simulink model "PVHome"  (R2022b)
settings: Solver=FixedStepDiscrete  StartTime=0.0  StopTime=2  FixedStep=5e-6  RelTol=1e-3
undefined symbols (not defined in the file): Ion, Lithium
libraries: spsSeriesRLCBranchLib x175, spsBreakerLib x103, spsPWMGeneratorDCDCLib x94, spsThyristorLib x78, slpidlib x72, spsIGBTDiodeLib x62, spsThreePhaseVIMeasurementLib x59, spsThreePhaseBreakerLib x45, spsVoltageMeasurementLib x45, spsDiodeLib x39, spsThreePhaseParallelRLCBranchLib x38, spsMosfetLib x32
(part 15 of 16)

== matlab function PVHome/Subsystem6/Centralized System ==
  data: H1_Pv_Breaker output; P_Pv input; Bi_B_Charge_Breaker_Buck output; Bi_B_Charge_Breaker_Boost output; H1_Grid_Breaker output; H1_Grid_Circuit_Breaker output; P_load input; Bi_B_Breaker_Discharge_Boost output; Bi_B_Breaker_Discharge_Buck output; H1_B_Ground_Discharge output; SOCbH1 input; Grid_Energy_Trading_Breaker output; Wind_Breaker_Boost output; P_Wind input; P_Real_Grid input; Wind_Breaker_Buck output; V_PV_1 input; V_Wind input; Wind_Power_Battery_Breaker_Boost output; Wind_Power_Battery_Breaker_Buck output; Battery_Passing_Voltage input; P1_C1 output
function [H1_Pv_Breaker, Bi_B_Charge_Breaker_Buck,Bi_B_Charge_Breaker_Boost, H1_Grid_Breaker, H1_Grid_Circuit_Breaker,Bi_B_Breaker_Discharge_Boost, Bi_B_Breaker_Discharge_Buck, H1_B_Ground_Discharge, Grid_Energy_Trading_Breaker, Wind_Breaker_Boost, Wind_Breaker_Buck, Wind_Power_Battery_Breaker_Boost, Wind_Power_Battery_Breaker_Buck, P1_C1] = control_logic(P_Pv, P_load, SOCbH1, P_Wind, P_Real_Grid, V_PV_1, V_Wind, Battery_Passing_Voltage)

% Make positive
P_Pv   = abs(P_Pv);
P_load = abs(P_load);
SOCbH1 = abs(SOCbH1);
P_Wind = abs(P_Wind);
V_PV_1 = abs(V_PV_1);
V_Wind = abs(V_Wind);
Battery_Passing_Voltage = abs(Battery_Passing_Voltage);

eps = 1;

%% DEFAULT STATES

% DC Ideal Switches (1 = ON)
H1_Pv_Breaker = 0;
Bi_B_Charge_Breaker_Buck  = 0;
Bi_B_Charge_Breaker_Boost=0;
Bi_B_Breaker_Discharge_Boost=0;
Bi_B_Breaker_Discharge_Buck=0;
H1_B_Ground_Discharge=0;
Wind_Breaker_Boost=0;
Wind_Breaker_Buck=0;
Wind_Power_Battery_Breaker_Boost=0;
Wind_Power_Battery_Breaker_Buck=0;
P1_C1=0;

% AC Breakers (0 = CLOSED)
H1_Grid_Breaker = 1;  % default OPEN
H1_Grid_Circuit_Breaker = 1;  % default OPEN
Grid_Energy_Trading_Breaker=1; % default open



%% CASE 1: No PV and no Wind
if (P_Pv+ P_Wind) <= eps %eps=0.01 (almost 0)

    % DC OFF
    H1_Pv_Breaker = 0;
    Bi_B_Charge_Breaker_Buck  = 0;
    Bi_B_Breaker_Discharge_Boost=0;
    H1_B_Ground_Discharge=0;
    Bi_B_Breaker_Discharge_Buck=0;
    Wind_Breaker_Boost=0;
    Wind_Breaker_Buck=0;
    Wind_Power_Battery_Breaker_Boost=0;
    Wind_Power_Battery_Breaker_Buck=0;
    P1_C1=0;


    % AC CLOSED (use grid)
    H1_Grid_Breaker         = 0;
    H1_Grid_Circuit_Breaker = 1;
    Grid_Energy_Trading_Breaker=1; %energy trading window open


%% CASE 2: PV and wind > Load
elseif (P_Pv + P_Wind) > P_load

    % Use PV
    H1_Pv_Breaker = 1;
    H1_Grid_Breaker = 1;
    H1_Grid_Circuit_Breaker = 1;

    if (SOCbH1) < 90 % if the value of soc is between is less than 90%, the battery can charge
        
        Bi_B_Breaker_Discharge_Boost=0;
        Bi_B_Breaker_Discharge_Buck=0;
        H1_B_Ground_Discharge=0;
        Grid_Energy_Trading_Breaker=1;
        P1_C1=0;        

        if (V_PV_1 > V_Wind) %boosts up
            Wind_Power_Battery_Breaker_Boost=1;
            Wind_Power_Battery_Breaker_Buck=0;
            Wind_Breaker_Boost=1;
            Wind_Breaker_Buck=0;
            if (Battery_Passing_Voltage)>60
                Bi_B_Charge_Breaker_Buck=1;
                Bi_B_Charge_Breaker_Boost=0;
            elseif (Battery_Passing_Voltage<60)
                Bi_B_Charge_Breaker_Buck=0;
                Bi_B_Charge_Breaker_Boost=1;
            end

        elseif (V_PV_1 < V_Wind)
            Wind_Power_Battery_Breaker_Boost=0;
            Wind_Power_Battery_Breaker_Buck=1;
            Wind_Breaker_Boost=0;
            Wind_Breaker_Buck=1;
        
            if (Battery_Passing_Voltage)>60
                Bi_B_Charge_Breaker_Buck=1;
                Bi_B_Charge_Breaker_Boost=0;
            elseif (Battery_Passing_Voltage)<60
                Bi_B_Charge_Breaker_Buck=0;
                Bi_B_Charge_Breaker_Boost=1;
            end
        
        end

    elseif SOCbH1==90
        Bi_B_Charge_Breaker_Boost=0;
        Bi_B_Charge_Breaker_Buck = 0;
        Bi_B_Breaker_Discharge_Boost=0;
        Bi_B_Breaker_Discharge_Buck=0;
        H1_B_Ground_Discharge=0;
        Grid_Energy_Trading_Breaker=0; %the power is sold to grid
        P1_C1=1; %the power is sold to C1

        if (V_PV_1 > V_Wind) %boosts up
        Wind_Power_Battery_Breaker_Boost=1;
        Wind_Power_Battery_Breaker_Buck=0;
        Wind_Breaker_Boost=1;
        Wind_Breaker_Buck=0;
        if (Battery_Passing_Voltage)>60
            Bi_B_Charge_Breaker_Buck=1;
            Bi_B_Charge_Breaker_Boost=0;
        elseif (Battery_Passing_Voltage<60)
            Bi_B_Charge_Breaker_Buck=0;
            Bi_B_Charge_Breaker_Boost=1;
        end

    elseif (V_PV_1 < V_Wind)
        Wind_Power_Battery_Breaker_Boost=0;
        Wind_Power_Battery_Breaker_Buck=1;
        Wind_Breaker_Boost=0;
        Wind_Breaker_Buck=1;
        
        if (Battery_Passing_Voltage)>60
            Bi_B_Charge_Breaker_Buck=1;
            Bi_B_Charge_Breaker_Boost=0;
        elseif (Battery_Passing_Voltage)<60
            Bi_B_Charge_Breaker_Buck=0;
            Bi_B_Charge_Breaker_Boost=1;
        end
        end
    end



%% CASE 3: PV and wind < Load
elseif (P_Pv + P_Wind) < (P_load) && (H1_Grid_Breaker~=0) %open (1 means open)

    % Use PV
    H1_Pv_Breaker = 1;
    H1_Grid_Circuit_Breaker = 0;
    Grid_Energy_Trading_Breaker=1;      
    Bi_B_Charge_Breaker_Buck=0; %no charging
    Bi_B_Charge_Breaker_Boost=0; %no charging
    P1_C1=0;


    if (V_PV_1)>60
        Bi_B_Breaker_Discharge_Boost=1;
        Bi_B_Breaker_Discharge_Buck=0;
        H1_B_Ground_Discharge=1;
    elseif(V_PV_1)<60
        Bi_B_Breaker_Discharge_Boost=0;
        Bi_B_Breaker_Discharge_Buck=1;
        H1_B_Ground_Discharge=1;
    end

    if (V_PV_1 > V_Wind) %boosts up
        Wind_Power_Battery_Breaker_Boost=1;
        Wind_Power_Battery_Breaker_Buck=0;
        Wind_Breaker_Boost=1;
        Wind_Breaker_Buck=0;
        
    elseif (V_PV_1 < V_Wind)
        Wind_Power_Battery_Breaker_Boost=0;
        Wind_Power_Battery_Breaker_Buck=1;
        Wind_Breaker_Boost=0;
        Wind_Breaker_Buck=1;
    end 

    
   

           
%% CASE 4:
elseif (P_Pv + P_Wind) < (P_load) && (H1_Grid_Breaker~=1) %closed (0) (no charging)

        % Use PV
    H1_Pv_Breaker = 1;
    H1_Grid_Circuit_Breaker = 0;
    Grid_Energy_Trading_Breaker=1;      
    Bi_B_Charge_Breaker_Buck=0; %(no charging)
    Bi_B_Charge_Breaker_Boost=0; %(no charging)
    Bi_B_Breaker_Discharge_Boost=0;
    Bi_B_Breaker_Discharge_Buck=0;
    H1_B_Ground_Discharge=0;
    P1_C1=0;


    if (V_PV_1 > V_Wind) %boosts up
        Wind_Power_Battery_Breaker_Boost=1;
        Wind_Power_Battery_Breaker_Buck=0;
        Wind_Breaker_Boost=1;
        Wind_Breaker_Buck=0;
        
    elseif (V_PV_1 < V_Wind)
        Wind_Power_Battery_Breaker_Boost=0;
        Wind_Power_Battery_Breaker_Buck=1;
        Wind_Breaker_Boost=0;
        Wind_Breaker_Buck=1;
    end 


%% CASE 5:
elseif (P_Pv + P_Wind+ P_Real_Grid) < P_Load 
    % Use PV
    H1_Grid_Breaker=0;
    H1_Pv_Breaker = 1;
    H1_Grid_Circuit_Breaker = 0;
    Grid_Energy_Trading_Breaker=1;      
    Bi_B_Charge_Breaker_Buck=0; %(no charging)
    Bi_B_Charge_Breaker_Boost=0; %(no charging)
    P1_C1=0;

    %discharging
    if (V_PV_1)>60
        Bi_B_Breaker_Discharge_Boost=1;
        Bi_B_Breaker_Discharge_Buck=0;
        H1_B_Ground_Discharge=1;
    elseif(V_PV_1)<60
        Bi_B_Breaker_Discharge_Boost=0;
        Bi_B_Breaker_Discharge_Buck=1;
        H1_B_Ground_Discharge=1;
    end

    if (V_PV_1 > V_Wind) %boosts up
        Wind_Power_Battery_Breaker_Boost=1;
        Wind_Power_Battery_Breaker_Buck=0;
        Wind_Breaker_Boost=1;
        Wind_Breaker_Buck=0;
        
    elseif (V_PV_1 < V_Wind) %bucks down
        Wind_Power_Battery_Breaker_Boost=0;
        Wind_Power_Battery_Breaker_Buck=1;
        Wind_Breaker_Boost=0;
        Wind_Breaker_Buck=1;
    end 

end


end

== matlab function PVHome/Subsystem5/MATLAB Function9 ==
  data: V_PV_1 input; Wind_Breaker_Boost_Signal_Out output; Sixty input
function Wind_Breaker_Boost_Signal_Out = fcn(V_PV_1, Sixty)
V_PV_1 = abs(V_PV_1);
Sixty = abs(Sixty);

D=1-(V_PV_1/Sixty);
Wind_Breaker_Boost_Signal_Out = D; %Vout

== matlab function PVHome/Subsystem4/MATLAB Function2 ==
  data: x input; a output; ma input; shift_k input; b output; c output
function [a,b,c]=ref_generation(x,ma,shift_k)
a=(ma*(sin((x)+shift_k)));
b=(ma*(sin((x)+shift_k-(2*pi/3))));
c=(ma*(sin((x)+shift_k+(2*pi/3))));

%ma is modulation index
%x is wt rad/s
%shift_k is phase angle

== matlab function PVHome/Subsystem4/MATLAB Function3 ==
  data: u input; y output
function y = fcn(u)
% This will output 1 - u
y = 1 - u;

== matlab function PVHome/Subsystem4/MATLAB Function4 ==
  data: u input; y output
function y = fcn(u)
% This will output 1 - u
y = 1 - u;

== matlab function PVHome/Subsystem4/MATLAB Function6 ==
  data: u input; y output
function y = fcn(u)
% This will output 1 - u
y = 1 - u;

== matlab function PVHome/Subsystem4/MATLAB Function7 ==
  data: V_PV_1 input; Wind_Breaker_Boost_Signal_Out output; V_Wind input
function Wind_Breaker_Boost_Signal_Out = fcn(V_PV_1, V_Wind)
V_PV_1 = abs(V_PV_1);
V_Wind = abs(V_Wind);

D=1-(V_PV_1/V_Wind);
Wind_Breaker_Boost_Signal_Out = D; %Vout

== matlab function PVHome/Subsystem4/MATLAB Function8 ==
  data: Sixty input; Wind_Breaker_Boost_Signal_Out output; V_PV_1 input
function Wind_Breaker_Boost_Signal_Out = fcn(Sixty, V_PV_1)
Sixty = abs(Sixty);
V_PV_1 = abs(V_PV_1);

D=1-(Sixty/V_PV_1);
Wind_Breaker_Boost_Signal_Out = D; %Vout

== matlab function PVHome/Subsystem4/MATLAB Function9 ==
  data: V_PV_1 input; Wind_Breaker_Boost_Signal_Out output; Sixty input
function Wind_Breaker_Boost_Signal_Out = fcn(V_PV_1, Sixty)
V_PV_1 = abs(V_PV_1);
Sixty = abs(Sixty);

D=1-(V_PV_1/Sixty);
Wind_Breaker_Boost_Signal_Out = D; %Vout

== matlab function PVHome/Subsystem6/MATLAB Function2 ==
  data: x input; a output; ma input; shift_k input; b output; c output
function [a,b,c]=ref_generation(x,ma,shift_k)
a=(ma*(sin((x)+shift_k)));
b=(ma*(sin((x)+shift_k-(2*pi/3))));
c=(ma*(sin((x)+shift_k+(2*pi/3))));

%ma is modulation index
%x is wt rad/s
%shift_k is phase angle

== matlab function PVHome/Subsystem6/MATLAB Function3 ==
  data: u input; y output
function y = fcn(u)
% This will output 1 - u
y = 1 - u;

== matlab function PVHome/Subsystem6/MATLAB Function4 ==
  data: u input; y output
function y = fcn(u)
% This will output 1 - u
y = 1 - u;

== matlab function PVHome/Subsystem6/MATLAB Function6 ==
  data: u input; y output
function y = fcn(u)
% This will output 1 - u
y = 1 - u;

== matlab function PVHome/Subsystem6/MATLAB Function7 ==
  data: V_PV_1 input; Wind_Breaker_Boost_Signal_Out output; V_Wind input
function Wind_Breaker_Boost_Signal_Out = fcn(V_PV_1, V_Wind)
V_PV_1 = abs(V_PV_1);
V_Wind = abs(V_Wind);

D=1-(V_PV_1/V_Wind);
Wind_Breaker_Boost_Signal_Out = D; %Vout

== matlab function PVHome/Subsystem6/MATLAB Function8 ==
  data: Sixty input; Wind_Breaker_Boost_Signal_Out output; V_PV_1 input
function Wind_Breaker_Boost_Signal_Out = fcn(Sixty, V_PV_1)
Sixty = abs(Sixty);
V_PV_1 = abs(V_PV_1);

D=1-(Sixty/V_PV_1);
Wind_Breaker_Boost_Signal_Out = D; %Vout

== matlab function PVHome/Subsystem6/MATLAB Function9 ==
  data: V_PV_1 input; Wind_Breaker_Boost_Signal_Out output; Sixty input
function Wind_Breaker_Boost_Signal_Out = fcn(V_PV_1, Sixty)
V_PV_1 = abs(V_PV_1);
Sixty = abs(Sixty);

D=1-(V_PV_1/Sixty);
Wind_Breaker_Boost_Signal_Out = D; %Vout

== matlab function PVHome/Subsystem3/MATLAB Function2 ==
  data: x input; a output; ma input; shift_k input; b output; c output
function [a,b,c]=ref_generation(x,ma,shift_k)
a=(ma*(sin((x)+shift_k)));
b=(ma*(sin((x)+shift_k-(2*pi/3))));
c=(ma*(sin((x)+shift_k+(2*pi/3))));

%ma is modulation index
%x is wt rad/s
%shift_k is phase angle

== matlab function PVHome/Subsystem3/MATLAB Function3 ==
  data: u input; y output
function y = fcn(u)
% This will output 1 - u
y = 1 - u;

== matlab function PVHome/Subsystem3/MATLAB Function4 ==
  data: u input; y output
function y = fcn(u)
% This will output 1 - u
y = 1 - u;

== matlab function PVHome/Subsystem3/MATLAB Function6 ==
  data: u input; y output
function y = fcn(u)
% This will output 1 - u
y = 1 - u;

== matlab function PVHome/Subsystem3/MATLAB Function7 ==
  data: V_PV_1 input; Wind_Breaker_Boost_Signal_Out output; V_Wind input
function Wind_Breaker_Boost_Signal_Out = fcn(V_PV_1, V_Wind)
V_PV_1 = abs(V_PV_1);
V_Wind = abs(V_Wind);

D=1-(V_PV_1/V_Wind);
Wind_Breaker_Boost_Signal_Out = D; %Vout

== matlab function PVHome/Subsystem3/MATLAB Function8 ==
  data: Sixty input; Wind_Breaker_Boost_Signal_Out output; V_PV_1 input
function Wind_Breaker_Boost_Signal_Out = fcn(Sixty, V_PV_1)
Sixty = abs(Sixty);
V_PV_1 = abs(V_PV_1);

D=1-(Sixty/V_PV_1);
Wind_Breaker_Boost_Signal_Out = D; %Vout

== matlab function PVHome/Subsystem3/MATLAB Function9 ==
  data: V_PV_1 input; Wind_Breaker_Boost_Signal_Out output; Sixty input
function Wind_Breaker_Boost_Signal_Out = fcn(V_PV_1, Sixty)
V_PV_1 = abs(V_PV_1);
Sixty = abs(Sixty);

D=1-(V_PV_1/Sixty);
Wind_Breaker_Boost_Signal_Out = D; %Vout

== matlab function PVHome/Subsystem1/MATLAB Function2 ==
  data: x input; a output; ma input; shift_k input; b output; c output
function [a,b,c]=ref_generation(x,ma,shift_k)
a=(ma*(sin((x)+shift_k)));
b=(ma*(sin((x)+shift_k-(2*pi/3))));
c=(ma*(sin((x)+shift_k+(2*pi/3))));

%ma is modulation index
%x is wt rad/s
%shift_k is phase angle

== matlab function PVHome/Subsystem1/MATLAB Function3 ==
  data: u input; y output
function y = fcn(u)
% This will output 1 - u
y = 1 - u;

== matlab function PVHome/Subsystem1/MATLAB Function4 ==
  data: u input; y output
function y = fcn(u)
% This will output 1 - u
y = 1 - u;

== matlab function PVHome/Subsystem1/MATLAB Function6 ==
  data: u input; y output
function y = fcn(u)
% This will output 1 - u
y = 1 - u;

== matlab function PVHome/Subsystem1/MATLAB Function7 ==
  data: V_PV_1 input; Wind_Breaker_Boost_Signal_Out output; V_Wind input
function Wind_Breaker_Boost_Signal_Out = fcn(V_PV_1, V_Wind)
V_PV_1 = abs(V_PV_1);
V_Wind = abs(V_Wind);

D=1-(V_PV_1/V_Wind);
Wind_Breaker_Boost_Signal_Out = D; %Vout

== matlab function PVHome/Subsystem1/MATLAB Function8 ==
  data: Sixty input; Wind_Breaker_Boost_Signal_Out output; V_PV_1 input
function Wind_Breaker_Boost_Signal_Out = fcn(Sixty, V_PV_1)
Sixty = abs(Sixty);
V_PV_1 = abs(V_PV_1);

D=1-(Sixty/V_PV_1);
Wind_Breaker_Boost_Signal_Out = D; %Vout

== matlab function PVHome/Subsystem1/MATLAB Function9 ==
  data: V_PV_1 input; Wind_Breaker_Boost_Signal_Out output; Sixty input
function Wind_Breaker_Boost_Signal_Out = fcn(V_PV_1, Sixty)
V_PV_1 = abs(V_PV_1);
Sixty = abs(Sixty);

D=1-(V_PV_1/Sixty);
Wind_Breaker_Boost_Signal_Out = D; %Vout

== matlab function PVHome/Subsystem2/MATLAB Function4 ==
  data: u input; y output
function y = fcn(u)
% This will output 1 - u
y = 1 - u;

== matlab function PVHome/Subsystem2/MATLAB Function6 ==
  data: u input; y output
function y = fcn(u)
% This will output 1 - u
y = 1 - u;

== matlab function PVHome/Subsystem2/MATLAB Function7 ==
  data: V_PV_1 input; Wind_Breaker_Boost_Signal_Out output; V_Wind input
function Wind_Breaker_Boost_Signal_Out = fcn(V_PV_1, V_Wind)
V_PV_1 = abs(V_PV_1);
V_Wind = abs(V_Wind);

D=1-(V_PV_1/V_Wind);
Wind_Breaker_Boost_Signal_Out = D; %Vout

== matlab function PVHome/Subsystem2/MATLAB Function8 ==
  data: Sixty input; Wind_Breaker_Boost_Signal_Out output; V_PV_1 input
function Wind_Breaker_Boost_Signal_Out = fcn(Sixty, V_PV_1)
Sixty = abs(Sixty);
V_PV_1 = abs(V_PV_1);

D=1-(Sixty/V_PV_1);
Wind_Breaker_Boost_Signal_Out = D; %Vout

== matlab function PVHome/Subsystem2/MATLAB Function9 ==
  data: V_PV_1 input; Wind_Breaker_Boost_Signal_Out output; Sixty input
function Wind_Breaker_Boost_Signal_Out = fcn(V_PV_1, Sixty)
V_PV_1 = abs(V_PV_1);
Sixty = abs(Sixty);

D=1-(V_PV_1/Sixty);
Wind_Breaker_Boost_Signal_Out = D; %Vout

== matlab function PVHome/Subsystem6/MATLAB Function ==
  data: V_PV input; duty output; I_PV input; deltaD input
function duty = mppt_pno(V_PV, I_PV, deltaD)

persistent prevP prevDuty

if isempty(prevP)
    prevP = 0;
    prevDuty = 0.5;   % Start at 50%
end

% Current PV power
P = V_PV * I_PV;

% Basic P&O
if P > prevP
    prevDuty = prevDuty + deltaD;
else
    prevDuty = prevDuty - deltaD;
end

% Safe duty limits for boost converter
if prevDuty > 0.75
    prevDuty = 0.75;
elseif prevDuty < 0.10
    prevDuty = 0.10;
end

% Update previous power
prevP = P;

% Output duty
duty = prevDuty;

end

== matlab function PVHome/Subsystem2/MATLAB Local MPPT 2 ==
  data: V_PV_2 input; duty output; I_PV_2 input; deltaD_2 input
function duty = mppt_pno(V_PV_2, I_PV_2, deltaD_2)

persistent prevP prevDuty

if isempty(prevP)
    prevP = 0;
    prevDuty = 0.5;   % Start at 50%
end

% Current PV power
P = V_PV_2 * I_PV_2;

% Basic P&O
if P > prevP
    prevDuty = prevDuty + deltaD_2;
else
    prevDuty = prevDuty - deltaD_2;
end

% Safe duty limits for boost converter
if prevDuty > 0.75
    prevDuty = 0.75;
elseif prevDuty < 0.10
    prevDuty = 0.10;
end

% Update previous power
prevP = P;

% Output duty
duty = prevDuty;

end

== matlab function PVHome/Subsystem2/MATLAB Function10 ==
  data: V_PV_1 input; Wind_Breaker_Boost_Signal_Out output; V_Pv_2 input
function Wind_Breaker_Boost_Signal_Out = fcn(V_PV_1, V_Pv_2)
V_PV_1 = abs(V_PV_1);
V_Pv_2 = abs(V_Pv_2);

D=1-(V_PV_1/V_Pv_2);
Wind_Breaker_Boost_Signal_Out = D; %Vout

== matlab function PVHome/Subsystem2/MATLAB Function5 ==
  data: u input; y output
function y = fcn(u)
% This will output 1 - u
y = 1 - u;

== matlab function PVHome/Subsystem3/MATLAB Function5 ==
  data: Fault_Signal output; I_Fault input
function Fault_Signal = fcn(I_Fault)

I_Fault = abs(I_Fault)

Fault_Signal=0; %closed

if I_Fault>30
    Fault_Signal=1;
elseif I_Fault<30
    Fault_Signal=0;
end

== matlab function PVHome/Subsystem4/MATLAB Function5 ==
  data: Fault_Signal output; I_Fault input
function Fault_Signal = fcn(I_Fault)

I_Fault = abs(I_Fault)

Fault_Signal=0; %closed

if I_Fault>30
    Fault_Signal=1;
elseif I_Fault<30
    Fault_Signal=0;
end

== matlab function PVHome/Subsystem5/MATLAB Function5 ==
  data: Fault_Signal output; I_Fault input
function Fault_Signal = fcn(I_Fault)

I_Fault = abs(I_Fault)

Fault_Signal=0; %closed

if I_Fault>30
    Fault_Signal=1;
elseif I_Fault<30
    Fault_Signal=0;
end

== matlab function PVHome/Subsystem6/MATLAB Function5 ==
  data: Fault_Signal output; I_Fault input
function Fault_Signal = fcn(I_Fault)

I_Fault = abs(I_Fault)

Fault_Signal=0; %closed

if I_Fault>30
    Fault_Signal=1;
elseif I_Fault<30
    Fault_Signal=0;
end

== matlab function PVHome/Subsystem3/Subsystem/MATLAB Function10 ==
  data: x input; a output; ma input; shift_k input; b output; c output
function [a,b,c]=ref_generation(x,ma,shift_k)
a=(ma*(sin((x)+shift_k)));
b=(ma*(sin((x)+shift_k-(2*pi/3))));
c=(ma*(sin((x)+shift_k+(2*pi/3))));

%ma is modulation index
%x is wt rad/s
%shift_k is phase angle

== matlab function PVHome/Subsystem3/Subsystem/MATLAB Function11 ==
  data: u input; y output
function y = fcn(u)
% This will output 1 - u
y = 1 - u;

== matlab function PVHome/Subsystem3/Subsystem/MATLAB Function12 ==
  data: V_PV_1 input; Wind_Breaker_Boost_Signal_Out output; Sixty input
function Wind_Breaker_Boost_Signal_Out = fcn(V_PV_1, Sixty)
V_PV_1 = abs(V_PV_1);
Sixty = abs(Sixty);

D=1-(V_PV_1/Sixty);
Wind_Breaker_Boost_Signal_Out = D; %Vout

== matlab function PVHome/Subsystem3/Subsystem/MATLAB Function5 ==
  data: SOCbHC1 input; V_Consumer_Battery_Boost_Breaker_Grid output; V_Consumer_Battery_Buck_Breaker_Grid output; Grid_Battery_Switch output; V_PV_1 input; V_Coming_Voltage_To_Battery input; P1_C1 input; Load input; P_Real_Grid_C1 input; H1_Battery_Discharge output; Buck_From_The_Excess_Prosumer_Breaker output; Boost_From_The_Excess_Prosumer_Breaker output; V_Consumer_Battery input; P1_C1_Excess_C1_Control output
function [V_Consumer_Battery_Boost_Breaker_Grid,V_Consumer_Battery_Buck_Breaker_Grid, Grid_Battery_Switch, H1_Battery_Discharge, Buck_From_The_Excess_Prosumer_Breaker, Boost_From_The_Excess_Prosumer_Breaker, P1_C1_Excess_C1_Control] = fcn(SOCbHC1, V_PV_1, V_Coming_Voltage_To_Battery, P1_C1,Load, P_Real_Grid_C1, V_Consumer_Battery)


SOCbHC1 = abs(SOCbHC1);
V_PV_1 = abs(V_PV_1);
V_Consumer_Battery = abs(V_Consumer_Battery);
V_Coming_Voltage_To_Battery = abs(V_Coming_Voltage_To_Battery);
%V_Coming_Voltage_To_Battery will be equal to V_PV_1
P_Real_Grid_C1 = abs(P_Real_Grid_C1);

%%Default States
V_Consumer_Battery_Boost_Breaker_Grid=0;
V_Consumer_Battery_Buck_Breaker_Grid=0;
Grid_Battery_Switch=0; % AC switch, always closed. 0 means closed in here.
H1_Battery_Discharge=0;
Buck_From_The_Excess_Prosumer_Breaker=0;
Boost_From_The_Excess_Prosumer_Breaker=0;
P1_C1_Excess_C1_Control=0;

%%Case 1: Charge

if (SOCbHC1)<=90
    Grid_Battery_Switch=0;
    if (V_Consumer_Battery)>60
        V_Consumer_Battery_Buck_Breaker_Grid=1;
        V_Consumer_Battery_Boost_Breaker_Grid=0;
    elseif (V_Consumer_Battery)<60
        V_Consumer_Battery_Buck_Breaker_Grid=0;
        V_Consumer_Battery_Boost_Breaker_Grid=1;
    end

    if (P1_C1)==1 && (V_Coming_Voltage_To_Battery)>5
        P1_C1_Excess_C1_Control=1;
        if (V_Coming_Voltage_To_Battery)>60
            Buck_From_The_Excess_Prosumer_Breaker=1;
            Boost_From_The_Excess_Prosumer_Breaker=0;
        elseif (V_Coming_Voltage_To_Battery)<60
            Buck_From_The_Excess_Prosumer_Breaker=0;
            Boost_From_The_Excess_Prosumer_Breaker=1;
        end
    elseif (P1_C1)==0 && (V_Coming_Voltage_To_Battery)<5
        Buck_From_The_Excess_Prosumer_Breaker=0;
        Boost_From_The_Excess_Prosumer_Breaker=0;
        P1_C1_Excess_C1_Control=0;
    end

elseif (SOCbHC1)==90
    V_Consumer_Battery_Boost_Breaker_Grid=0;
    V_Consumer_Battery_Buck_Breaker_Grid=0;
    Grid_Battery_Switch=1;
    H1_Battery_Discharge=0;
    Buck_From_The_Excess_Prosumer_Breaker=0;
    Boost_From_The_Excess_Prosumer_Breaker=0;
    P1_C1_Excess_C1_Control=0;
end

%%Case 2 Discharge

if (Load> P_Real_Grid_C1) || P_Real_Grid_C1<100
    V_Consumer_Battery_Boost_Breaker_Grid=0;
    V_Consumer_Battery_Buck_Breaker_Grid=0;
    Grid_Battery_Switch=1; 
    H1_Battery_Discharge=1;
    Buck_From_The_Excess_Prosumer_Breaker=0;
    Boost_From_The_Excess_Prosumer_Breaker=0;
    P1_C1_Excess_C1_Control=0;
end

== matlab function PVHome/Subsystem1/Centralized System ==
  data: H1_Pv_Breaker output; P_Pv input; Bi_B_Charge_Breaker_Buck output; Bi_B_Charge_Breaker_Boost output; H1_Grid_Breaker output; H1_Grid_Circuit_Breaker output; P_load input; Bi_B_Breaker_Discharge_Boost output; Bi_B_Breaker_Discharge_Buck output; H1_B_Ground_Discharge output; SOCbH1 input; Grid_Energy_Trading_Breaker output; Wind_Breaker_Boost output; P_Wind input; P_Real_Grid input; Wind_Breaker_Buck output; V_PV_1 input; V_Wind input; Wind_Power_Battery_Breaker_Boost output; Wind_Power_Battery_Breaker_Buck output; Battery_Passing_Voltage input; P1_C1 output
function [H1_Pv_Breaker, Bi_B_Charge_Breaker_Buck,Bi_B_Charge_Breaker_Boost, H1_Grid_Breaker, H1_Grid_Circuit_Breaker,Bi_B_Breaker_Discharge_Boost, Bi_B_Breaker_Discharge_Buck, H1_B_Ground_Discharge, Grid_Energy_Trading_Breaker, Wind_Breaker_Boost, Wind_Breaker_Buck, Wind_Power_Battery_Breaker_Boost, Wind_Power_Battery_Breaker_Buck, P1_C1] = control_logic(P_Pv, P_load, SOCbH1, P_Wind, P_Real_Grid, V_PV_1, V_Wind, Battery_Passing_Voltage)

% Make positive
P_Pv   = abs(P_Pv);
P_load = abs(P_load);
SOCbH1 = abs(SOCbH1);
P_Wind = abs(P_Wind);
V_PV_1 = abs(V_PV_1);
V_Wind = abs(V_Wind);
Battery_Passing_Voltage = abs(Battery_Passing_Voltage);

eps = 1;

%% DEFAULT STATES

% DC Ideal Switches (1 = ON)
H1_Pv_Breaker = 0;
Bi_B_Charge_Breaker_Buck  = 0;
Bi_B_Charge_Breaker_Boost=0;
Bi_B_Breaker_Discharge_Boost=0;
Bi_B_Breaker_Discharge_Buck=0;
H1_B_Ground_Discharge=0;
Wind_Breaker_Boost=0;
Wind_Breaker_Buck=0;
Wind_Power_Battery_Breaker_Boost=0;
Wind_Power_Battery_Breaker_Buck=0;
P1_C1=0;

% AC Breakers (0 = CLOSED)
H1_Grid_Breaker = 1;  % default OPEN
H1_Grid_Circuit_Breaker = 1;  % default OPEN
Grid_Energy_Trading_Breaker=1; % default open



%% CASE 1: No PV and no Wind
if (P_Pv+ P_Wind) <= eps %eps=0.01 (almost 0)

    % DC OFF
    H1_Pv_Breaker = 0;
    Bi_B_Charge_Breaker_Buck  = 0;
    Bi_B_Breaker_Discharge_Boost=0;
    H1_B_Ground_Discharge=0;
    Bi_B_Breaker_Discharge_Buck=0;
    Wind_Breaker_Boost=0;
    Wind_Breaker_Buck=0;
    Wind_Power_Battery_Breaker_Boost=0;
    Wind_Power_Battery_Breaker_Buck=0;
    P1_C1=0;


    % AC CLOSED (use grid)
    H1_Grid_Breaker         = 0;
    H1_Grid_Circuit_Breaker = 1;
    Grid_Energy_Trading_Breaker=1; %energy trading window open


%% CASE 2: PV and wind > Load
elseif (P_Pv + P_Wind) > P_load

    % Use PV
    H1_Pv_Breaker = 1;
    H1_Grid_Breaker = 1;
    H1_Grid_Circuit_Breaker = 1;

    if (SOCbH1) < 90 % if the value of soc is between is less than 90%, the battery can charge
        
        Bi_B_Breaker_Discharge_Boost=0;
        Bi_B_Breaker_Discharge_Buck=0;
        H1_B_Ground_Discharge=0;
        Grid_Energy_Trading_Breaker=1;
        P1_C1=0;        

        if (V_PV_1 > V_Wind) %boosts up
            Wind_Power_Battery_Breaker_Boost=1;
            Wind_Power_Battery_Breaker_Buck=0;
            Wind_Breaker_Boost=1;
            Wind_Breaker_Buck=0;
            if (Battery_Passing_Voltage)>60
                Bi_B_Charge_Breaker_Buck=1;
                Bi_B_Charge_Breaker_Boost=0;
            elseif (Battery_Passing_Voltage<60)
                Bi_B_Charge_Breaker_Buck=0;
                Bi_B_Charge_Breaker_Boost=1;
            end

        elseif (V_PV_1 < V_Wind)
            Wind_Power_Battery_Breaker_Boost=0;
            Wind_Power_Battery_Breaker_Buck=1;
            Wind_Breaker_Boost=0;
            Wind_Breaker_Buck=1;
        
            if (Battery_Passing_Voltage)>60
                Bi_B_Charge_Breaker_Buck=1;
                Bi_B_Charge_Breaker_Boost=0;
            elseif (Battery_Passing_Voltage)<60
                Bi_B_Charge_Breaker_Buck=0;
                Bi_B_Charge_Breaker_Boost=1;
            end
        
        end

    elseif SOCbH1==90
        Bi_B_Charge_Breaker_Boost=0;
        Bi_B_Charge_Breaker_Buck = 0;
        Bi_B_Breaker_Discharge_Boost=0;
        Bi_B_Breaker_Discharge_Buck=0;
        H1_B_Ground_Discharge=0;
        Grid_Energy_Trading_Breaker=0; %the power is sold to grid
        P1_C1=1; %the power is sold to C1

        if (V_PV_1 > V_Wind) %boosts up
        Wind_Power_Battery_Breaker_Boost=1;
        Wind_Power_Battery_Breaker_Buck=0;
        Wind_Breaker_Boost=1;
        Wind_Breaker_Buck=0;
        if (Battery_Passing_Voltage)>60
            Bi_B_Charge_Breaker_Buck=1;
            Bi_B_Charge_Breaker_Boost=0;
        elseif (Battery_Passing_Voltage<60)
            Bi_B_Charge_Breaker_Buck=0;
            Bi_B_Charge_Breaker_Boost=1;
        end

    elseif (V_PV_1 < V_Wind)
        Wind_Power_Battery_Breaker_Boost=0;
        Wind_Power_Battery_Breaker_Buck=1;
        Wind_Breaker_Boost=0;
        Wind_Breaker_Buck=1;
        
        if (Battery_Passing_Voltage)>60
            Bi_B_Charge_Breaker_Buck=1;
            Bi_B_Charge_Breaker_Boost=0;
        elseif (Battery_Passing_Voltage)<60
            Bi_B_Charge_Breaker_Buck=0;
            Bi_B_Charge_Breaker_Boost=1;
        end
        end
    end



%% CASE 3: PV and wind < Load
elseif (P_Pv + P_Wind) < (P_load) && (H1_Grid_Breaker~=0) %open (1 means open)

    % Use PV
    H1_Pv_Breaker = 1;
    H1_Grid_Circuit_Breaker = 0;
    Grid_Energy_Trading_Breaker=1;      
    Bi_B_Charge_Breaker_Buck=0; %no charging
    Bi_B_Charge_Breaker_Boost=0; %no charging
    P1_C1=0;


    if (V_PV_1)>60
        Bi_B_Breaker_Discharge_Boost=1;
        Bi_B_Breaker_Discharge_Buck=0;
        H1_B_Ground_Discharge=1;
    elseif(V_PV_1)<60
        Bi_B_Breaker_Discharge_Boost=0;
        Bi_B_Breaker_Discharge_Buck=1;
        H1_B_Ground_Discharge=1;
    end

    if (V_PV_1 > V_Wind) %boosts up
        Wind_Power_Battery_Breaker_Boost=1;
        Wind_Power_Battery_Breaker_Buck=0;
        Wind_Breaker_Boost=1;
        Wind_Breaker_Buck=0;
        
    elseif (V_PV_1 < V_Wind)
        Wind_Power_Battery_Breaker_Boost=0;
        Wind_Power_Battery_Breaker_Buck=1;
        Wind_Breaker_Boost=0;
        Wind_Breaker_Buck=1;
    end 

    
   

           
%% CASE 4:
elseif (P_Pv + P_Wind) < (P_load) && (H1_Grid_Breaker~=1) %closed (0) (no charging)

        % Use PV
    H1_Pv_Breaker = 1;
    H1_Grid_Circuit_Breaker = 0;
    Grid_Energy_Trading_Breaker=1;      
    Bi_B_Charge_Breaker_Buck=0; %(no charging)
    Bi_B_Charge_Breaker_Boost=0; %(no charging)
    Bi_B_Breaker_Discharge_Boost=0;
    Bi_B_Breaker_Discharge_Buck=0;
    H1_B_Ground_Discharge=0;
    P1_C1=0;


    if (V_PV_1 > V_Wind) %boosts up
        Wind_Power_Battery_Breaker_Boost=1;
        Wind_Power_Battery_Breaker_Buck=0;
        Wind_Breaker_Boost=1;
        Wind_Breaker_Buck=0;
        
    elseif (V_PV_1 < V_Wind)
        Wind_Power_Battery_Breaker_Boost=0;
        Wind_Power_Battery_Breaker_Buck=1;
        Wind_Breaker_Boost=0;
        Wind_Breaker_Buck=1;
    end 


%% CASE 5:
elseif (P_Pv + P_Wind+ P_Real_Grid) < P_Load 
    % Use PV
    H1_Grid_Breaker=0;
    H1_Pv_Breaker = 1;
    H1_Grid_Circuit_Breaker = 0;
    Grid_Energy_Trading_Breaker=1;      
    Bi_B_Charge_Breaker_Buck=0; %(no charging)
    Bi_B_Charge_Breaker_Boost=0; %(no charging)
    P1_C1=0;

    %discharging
    if (V_PV_1)>60
        Bi_B_Breaker_Discharge_Boost=1;
        Bi_B_Breaker_Discharge_Buck=0;
        H1_B_Ground_Discharge=1;
    elseif(V_PV_1)<60
        Bi_B_Breaker_Discharge_Boost=0;
        Bi_B_Breaker_Discharge_Buck=1;
        H1_B_Ground_Discharge=1;
    end

    if (V_PV_1 > V_Wind) %boosts up
        Wind_Power_Battery_Breaker_Boost=1;
        Wind_Power_Battery_Breaker_Buck=0;
        Wind_Breaker_Boost=1;
        Wind_Breaker_Buck=0;
        
    elseif (V_PV_1 < V_Wind) %bucks down
        Wind_Power_Battery_Breaker_Boost=0;
        Wind_Power_Battery_Breaker_Buck=1;
        Wind_Breaker_Boost=0;
        Wind_Breaker_Buck=1;
    end 

end


end

== matlab function PVHome/Subsystem1/Subsystem/MATLAB Function10 ==
  data: x input; a output; ma input; shift_k input; b output; c output
function [a,b,c]=ref_generation(x,ma,shift_k)
a=(ma*(sin((x)+shift_k)));
b=(ma*(sin((x)+shift_k-(2*pi/3))));
c=(ma*(sin((x)+shift_k+(2*pi/3))));

%ma is modulation index
%x is wt rad/s
%shift_k is phase angle

== matlab function PVHome/Subsystem1/Subsystem/MATLAB Function11 ==
  data: u input; y output
function y = fcn(u)
% This will output 1 - u
y = 1 - u;

== matlab function PVHome/Subsystem1/Subsystem/MATLAB Function12 ==
  data: V_PV_1 input; Wind_Breaker_Boost_Signal_Out output; Sixty input
function Wind_Breaker_Boost_Signal_Out = fcn(V_PV_1, Sixty)
V_PV_1 = abs(V_PV_1);
Sixty = abs(Sixty);

D=1-(V_PV_1/Sixty);
Wind_Breaker_Boost_Signal_Out = D; %Vout

== matlab function PVHome/Subsystem1/Subsystem/MATLAB Function5 ==
  data: SOCbHC1 input; V_Consumer_Battery_Boost_Breaker_Grid output; V_Consumer_Battery_Buck_Breaker_Grid output; Grid_Battery_Switch output; V_PV_1 input; V_Coming_Voltage_To_Battery input; P1_C1 input; Load input; P_Real_Grid_C1 input; H1_Battery_Discharge output; Buck_From_The_Excess_Prosumer_Breaker output; Boost_From_The_Excess_Prosumer_Breaker output; V_Consumer_Battery input; P1_C1_Excess_C1_Control output
function [V_Consumer_Battery_Boost_Breaker_Grid,V_Consumer_Battery_Buck_Breaker_Grid, Grid_Battery_Switch, H1_Battery_Discharge, Buck_From_The_Excess_Prosumer_Breaker, Boost_From_The_Excess_Prosumer_Breaker, P1_C1_Excess_C1_Control] = fcn(SOCbHC1, V_PV_1, V_Coming_Voltage_To_Battery, P1_C1,Load, P_Real_Grid_C1, V_Consumer_Battery)


SOCbHC1 = abs(SOCbHC1);
V_PV_1 = abs(V_PV_1);
V_Consumer_Battery = abs(V_Consumer_Battery);
V_Coming_Voltage_To_Battery = abs(V_Coming_Voltage_To_Battery);
%V_Coming_Voltage_To_Battery will be equal to V_PV_1
P_Real_Grid_C1 = abs(P_Real_Grid_C1);

%%Default States
V_Consumer_Battery_Boost_Breaker_Grid=0;
V_Consumer_Battery_Buck_Breaker_Grid=0;
Grid_Battery_Switch=0; % AC switch, always closed. 0 means closed in here.
H1_Battery_Discharge=0;
Buck_From_The_Excess_Prosumer_Breaker=0;
Boost_From_The_Excess_Prosumer_Breaker=0;
P1_C1_Excess_C1_Control=0;

%%Case 1: Charge

if (SOCbHC1)<=90
    Grid_Battery_Switch=0;
    if (V_Consumer_Battery)>60
        V_Consumer_Battery_Buck_Breaker_Grid=1;
        V_Consumer_Battery_Boost_Breaker_Grid=0;
    elseif (V_Consumer_Battery)<60
        V_Consumer_Battery_Buck_Breaker_Grid=0;
        V_Consumer_Battery_Boost_Breaker_Grid=1;
    end

    if (P1_C1)==1 && (V_Coming_Voltage_To_Battery)>5
        P1_C1_Excess_C1_Control=1;
        if (V_Coming_Voltage_To_Battery)>60
            Buck_From_The_Excess_Prosumer_Breaker=1;
            Boost_From_The_Excess_Prosumer_Breaker=0;
        elseif (V_Coming_Voltage_To_Battery)<60
            Buck_From_The_Excess_Prosumer_Breaker=0;
            Boost_From_The_Excess_Prosumer_Breaker=1;
        end
    elseif (P1_C1)==0 && (V_Coming_Voltage_To_Battery)<5
        Buck_From_The_Excess_Prosumer_Breaker=0;
        Boost_From_The_Excess_Prosumer_Breaker=0;
        P1_C1_Excess_C1_Control=0;
    end

elseif (SOCbHC1)==90
    V_Consumer_Battery_Boost_Breaker_Grid=0;
    V_Consumer_Battery_Buck_Breaker_Grid=0;
    Grid_Battery_Switch=1;
    H1_Battery_Discharge=0;
    Buck_From_The_Excess_Prosumer_Breaker=0;
    Boost_From_The_Excess_Prosumer_Breaker=0;
    P1_C1_Excess_C1_Control=0;
end

%%Case 2 Discharge

if (Load> P_Real_Grid_C1) || P_Real_Grid_C1<100
    V_Consumer_Battery_Boost_Breaker_Grid=0;
    V_Consumer_Battery_Buck_Breaker_Grid=0;
    Grid_Battery_Switch=1; 
    H1_Battery_Discharge=1;
    Buck_From_The_Excess_Prosumer_Breaker=0;
    Boost_From_The_Excess_Prosumer_Breaker=0;
    P1_C1_Excess_C1_Control=0;
end

== matlab function PVHome/Subsystem6/Subsystem/MATLAB Function10 ==
  data: x input; a output; ma input; shift_k input; b output; c output
function [a,b,c]=ref_generation(x,ma,shift_k)
a=(ma*(sin((x)+shift_k)));
b=(ma*(sin((x)+shift_k-(2*pi/3))));
c=(ma*(sin((x)+shift_k+(2*pi/3))));

%ma is modulation index
%x is wt rad/s
%shift_k is phase angle

== matlab function PVHome/Subsystem6/Subsystem/MATLAB Function11 ==
  data: u input; y output
function y = fcn(u)
% This will output 1 - u
y = 1 - u;

== matlab function PVHome/Subsystem6/Subsystem/MATLAB Function12 ==
  data: V_PV_1 input; Wind_Breaker_Boost_Signal_Out output; Sixty input
function Wind_Breaker_Boost_Signal_Out = fcn(V_PV_1, Sixty)
V_PV_1 = abs(V_PV_1);
Sixty = abs(Sixty);

D=1-(V_PV_1/Sixty);
Wind_Breaker_Boost_Signal_Out = D; %Vout

== matlab function PVHome/Subsystem6/Subsystem/MATLAB Function5 ==
  data: SOCbHC1 input; V_Consumer_Battery_Boost_Breaker_Grid output; V_Consumer_Battery_Buck_Breaker_Grid output; Grid_Battery_Switch output; V_PV_1 input; V_Coming_Voltage_To_Battery input; P1_C1 input; Load input; P_Real_Grid_C1 input; H1_Battery_Discharge output; Buck_From_The_Excess_Prosumer_Breaker output; Boost_From_The_Excess_Prosumer_Breaker output; V_Consumer_Battery input; P1_C1_Excess_C1_Control output
function [V_Consumer_Battery_Boost_Breaker_Grid,V_Consumer_Battery_Buck_Breaker_Grid, Grid_Battery_Switch, H1_Battery_Discharge, Buck_From_The_Excess_Prosumer_Breaker, Boost_From_The_Excess_Prosumer_Breaker, P1_C1_Excess_C1_Control] = fcn(SOCbHC1, V_PV_1, V_Coming_Voltage_To_Battery, P1_C1,Load, P_Real_Grid_C1, V_Consumer_Battery)


SOCbHC1 = abs(SOCbHC1);
V_PV_1 = abs(V_PV_1);
V_Consumer_Battery = abs(V_Consumer_Battery);
V_Coming_Voltage_To_Battery = abs(V_Coming_Voltage_To_Battery);
%V_Coming_Voltage_To_Battery will be equal to V_PV_1
P_Real_Grid_C1 = abs(P_Real_Grid_C1);

%%Default States
V_Consumer_Battery_Boost_Breaker_Grid=0;
V_Consumer_Battery_Buck_Breaker_Grid=0;
Grid_Battery_Switch=0; % AC switch, always closed. 0 means closed in here.
H1_Battery_Discharge=0;
Buck_From_The_Excess_Prosumer_Breaker=0;
Boost_From_The_Excess_Prosumer_Breaker=0;
P1_C1_Excess_C1_Control=0;

%%Case 1: Charge

if (SOCbHC1)<=90
    Grid_Battery_Switch=0;
    if (V_Consumer_Battery)>60
        V_Consumer_Battery_Buck_Breaker_Grid=1;
        V_Consumer_Battery_Boost_Breaker_Grid=0;
    elseif (V_Consumer_Battery)<60
        V_Consumer_Battery_Buck_Breaker_Grid=0;
        V_Consumer_Battery_Boost_Breaker_Grid=1;
    end

    if (P1_C1)==1 && (V_Coming_Voltage_To_Battery)>5
        P1_C1_Excess_C1_Control=1;
        if (V_Coming_Voltage_To_Battery)>60
            Buck_From_The_Excess_Prosumer_Breaker=1;
            Boost_From_The_Excess_Prosumer_Breaker=0;
        elseif (V_Coming_Voltage_To_Battery)<60
            Buck_From_The_Excess_Prosumer_Breaker=0;
            Boost_From_The_Excess_Prosumer_Breaker=1;
        end
    elseif (P1_C1)==0 && (V_Coming_Voltage_To_Battery)<5
        Buck_From_The_Excess_Prosumer_Breaker=0;
        Boost_From_The_Excess_Prosumer_Breaker=0;
        P1_C1_Excess_C1_Control=0;
    end

elseif (SOCbHC1)==90
    V_Consumer_Battery_Boost_Breaker_Grid=0;
    V_Consumer_Battery_Buck_Breaker_Grid=0;
    Grid_Battery_Switch=1;
    H1_Battery_Discharge=0;
    Buck_From_The_Excess_Prosumer_Breaker=0;
    Boost_From_The_Excess_Prosumer_Breaker=0;
    P1_C1_Excess_C1_Control=0;
end

%%Case 2 Discharge

if (Load> P_Real_Grid_C1) || P_Real_Grid_C1<100
    V_Consumer_Battery_Boost_Breaker_Grid=0;
    V_Consumer_Battery_Buck_Breaker_Grid=0;
    Grid_Battery_Switch=1; 
    H1_Battery_Discharge=1;
    Buck_From_The_Excess_Prosumer_Breaker=0;
    Boost_From_The_Excess_Prosumer_Breaker=0;
    P1_C1_Excess_C1_Control=0;
end

== matlab function PVHome/Subsystem4/Subsystem/MATLAB Function10 ==
  data: x input; a output; ma input; shift_k input; b output; c output
function [a,b,c]=ref_generation(x,ma,shift_k)
a=(ma*(sin((x)+shift_k)));
b=(ma*(sin((x)+shift_k-(2*pi/3))));
c=(ma*(sin((x)+shift_k+(2*pi/3))));

%ma is modulation index
%x is wt rad/s
%shift_k is phase angle

== matlab function PVHome/Subsystem4/Subsystem/MATLAB Function11 ==
  data: u input; y output
function y = fcn(u)
% This will output 1 - u
y = 1 - u;

== matlab function PVHome/Subsystem4/Subsystem/MATLAB Function12 ==
  data: V_PV_1 input; Wind_Breaker_Boost_Signal_Out output; Sixty input
function Wind_Breaker_Boost_Signal_Out = fcn(V_PV_1, Sixty)
V_PV_1 = abs(V_PV_1);
Sixty = abs(Sixty);

D=1-(V_PV_1/Sixty);
Wind_Breaker_Boost_Signal_Out = D; %Vout

== matlab function PVHome/Subsystem4/Subsystem/MATLAB Function5 ==
  data: SOCbHC1 input; V_Consumer_Battery_Boost_Breaker_Grid output; V_Consumer_Battery_Buck_Breaker_Grid output; Grid_Battery_Switch output; V_PV_1 input; V_Coming_Voltage_To_Battery input; P1_C1 input; Load input; P_Real_Grid_C1 input; H1_Battery_Discharge output; Buck_From_The_Excess_Prosumer_Breaker output; Boost_From_The_Excess_Prosumer_Breaker output; V_Consumer_Battery input; P1_C1_Excess_C1_Control output
function [V_Consumer_Battery_Boost_Breaker_Grid,V_Consumer_Battery_Buck_Breaker_Grid, Grid_Battery_Switch, H1_Battery_Discharge, Buck_From_The_Excess_Prosumer_Breaker, Boost_From_The_Excess_Prosumer_Breaker, P1_C1_Excess_C1_Control] = fcn(SOCbHC1, V_PV_1, V_Coming_Voltage_To_Battery, P1_C1,Load, P_Real_Grid_C1, V_Consumer_Battery)


SOCbHC1 = abs(SOCbHC1);
V_PV_1 = abs(V_PV_1);
V_Consumer_Battery = abs(V_Consumer_Battery);
V_Coming_Voltage_To_Battery = abs(V_Coming_Voltage_To_Battery);
%V_Coming_Voltage_To_Battery will be equal to V_PV_1
P_Real_Grid_C1 = abs(P_Real_Grid_C1);

%%Default States
V_Consumer_Battery_Boost_Breaker_Grid=0;
V_Consumer_Battery_Buck_Breaker_Grid=0;
Grid_Battery_Switch=0; % AC switch, always closed. 0 means closed in here.
H1_Battery_Discharge=0;
Buck_From_The_Excess_Prosumer_Breaker=0;
Boost_From_The_Excess_Prosumer_Breaker=0;
P1_C1_Excess_C1_Control=0;

%%Case 1: Charge

if (SOCbHC1)<=90
    Grid_Battery_Switch=0;
    if (V_Consumer_Battery)>60
        V_Consumer_Battery_Buck_Breaker_Grid=1;
        V_Consumer_Battery_Boost_Breaker_Grid=0;
    elseif (V_Consumer_Battery)<60
        V_Consumer_Battery_Buck_Breaker_Grid=0;
        V_Consumer_Battery_Boost_Breaker_Grid=1;
    end

    if (P1_C1)==1 && (V_Coming_Voltage_To_Battery)>5
        P1_C1_Excess_C1_Control=1;
        if (V_Coming_Voltage_To_Battery)>60
            Buck_From_The_Excess_Prosumer_Breaker=1;
            Boost_From_The_Excess_Prosumer_Breaker=0;
        elseif (V_Coming_Voltage_To_Battery)<60
            Buck_From_The_Excess_Prosumer_Breaker=0;
            Boost_From_The_Excess_Prosumer_Breaker=1;
        end
    elseif (P1_C1)==0 && (V_Coming_Voltage_To_Battery)<5
        Buck_From_The_Excess_Prosumer_Breaker=0;
        Boost_From_The_Excess_Prosumer_Breaker=0;
        P1_C1_Excess_C1_Control=0;
    end

elseif (SOCbHC1)==90
    V_Consumer_Battery_Boost_Breaker_Grid=0;
    V_Consumer_Battery_Buck_Breaker_Grid=0;
    Grid_Battery_Switch=1;
    H1_Battery_Discharge=0;
    Buck_From_The_Excess_Prosumer_Breaker=0;
    Boost_From_The_Excess_Prosumer_Breaker=0;
    P1_C1_Excess_C1_Control=0;
end

%%Case 2 Discharge

if (Load> P_Real_Grid_C1) || P_Real_Grid_C1<100
    V_Consumer_Battery_Boost_Breaker_Grid=0;
    V_Consumer_Battery_Buck_Breaker_Grid=0;
    Grid_Battery_Switch=1; 
    H1_Battery_Discharge=1;
    Buck_From_The_Excess_Prosumer_Breaker=0;
    Boost_From_The_Excess_Prosumer_Breaker=0;
    P1_C1_Excess_C1_Control=0;
end

== matlab function PVHome/Subsystem5/Subsystem/MATLAB Function10 ==
  data: x input; a output; ma input; shift_k input; b output; c output
function [a,b,c]=ref_generation(x,ma,shift_k)
a=(ma*(sin((x)+shift_k)));
b=(ma*(sin((x)+shift_k-(2*pi/3))));
c=(ma*(sin((x)+shift_k+(2*pi/3))));

%ma is modulation index
%x is wt rad/s
%shift_k is phase angle

== matlab function PVHome/Subsystem5/Subsystem/MATLAB Function11 ==
  data: u input; y output
function y = fcn(u)
% This will output 1 - u
y = 1 - u;

== matlab function PVHome/Subsystem5/Subsystem/MATLAB Function12 ==
  data: V_PV_1 input; Wind_Breaker_Boost_Signal_Out output; Sixty input
function Wind_Breaker_Boost_Signal_Out = fcn(V_PV_1, Sixty)
V_PV_1 = abs(V_PV_1);
Sixty = abs(Sixty);

D=1-(V_PV_1/Sixty);
Wind_Breaker_Boost_Signal_Out = D; %Vout

== matlab function PVHome/Subsystem5/Subsystem/MATLAB Function5 ==
  data: SOCbHC1 input; V_Consumer_Battery_Boost_Breaker_Grid output; V_Consumer_Battery_Buck_Breaker_Grid output; Grid_Battery_Switch output; V_PV_1 input; V_Coming_Voltage_To_Battery input; P1_C1 input; Load input; P_Real_Grid_C1 input; H1_Battery_Discharge output; Buck_From_The_Excess_Prosumer_Breaker output; Boost_From_The_Excess_Prosumer_Breaker output; V_Consumer_Battery input; P1_C1_Excess_C1_Control output
function [V_Consumer_Battery_Boost_Breaker_Grid,V_Consumer_Battery_Buck_Breaker_Grid, Grid_Battery_Switch, H1_Battery_Discharge, Buck_From_The_Excess_Prosumer_Breaker, Boost_From_The_Excess_Prosumer_Breaker, P1_C1_Excess_C1_Control] = fcn(SOCbHC1, V_PV_1, V_Coming_Voltage_To_Battery, P1_C1,Load, P_Real_Grid_C1, V_Consumer_Battery)


SOCbHC1 = abs(SOCbHC1);
V_PV_1 = abs(V_PV_1);
V_Consumer_Battery = abs(V_Consumer_Battery);
V_Coming_Voltage_To_Battery = abs(V_Coming_Voltage_To_Battery);
%V_Coming_Voltage_To_Battery will be equal to V_PV_1
P_Real_Grid_C1 = abs(P_Real_Grid_C1);

%%Default States
V_Consumer_Battery_Boost_Breaker_Grid=0;
V_Consumer_Battery_Buck_Breaker_Grid=0;
Grid_Battery_Switch=0; % AC switch, always closed. 0 means closed in here.
H1_Battery_Discharge=0;
Buck_From_The_Excess_Prosumer_Breaker=0;
Boost_From_The_Excess_Prosumer_Breaker=0;
P1_C1_Excess_C1_Control=0;

%%Case 1: Charge

if (SOCbHC1)<=90
    Grid_Battery_Switch=0;
    if (V_Consumer_Battery)>60
        V_Consumer_Battery_Buck_Breaker_Grid=1;
        V_Consumer_Battery_Boost_Breaker_Grid=0;
    elseif (V_Consumer_Battery)<60
        V_Consumer_Battery_Buck_Breaker_Grid=0;
        V_Consumer_Battery_Boost_Breaker_Grid=1;
    end

    if (P1_C1)==1 && (V_Coming_Voltage_To_Battery)>5
        P1_C1_Excess_C1_Control=1;
        if (V_Coming_Voltage_To_Battery)>60
            Buck_From_The_Excess_Prosumer_Breaker=1;
            Boost_From_The_Excess_Prosumer_Breaker=0;
        elseif (V_Coming_Voltage_To_Battery)<60
            Buck_From_The_Excess_Prosumer_Breaker=0;
            Boost_From_The_Excess_Prosumer_Breaker=1;
        end
    elseif (P1_C1)==0 && (V_Coming_Voltage_To_Battery)<5
        Buck_From_The_Excess_Prosumer_Breaker=0;
        Boost_From_The_Excess_Prosumer_Breaker=0;
        P1_C1_Excess_C1_Control=0;
    end

elseif (SOCbHC1)==90
    V_Consumer_Battery_Boost_Breaker_Grid=0;
    V_Consumer_Battery_Buck_Breaker_Grid=0;
    Grid_Battery_Switch=1;
    H1_Battery_Discharge=0;
    Buck_From_The_Excess_Prosumer_Breaker=0;
    Boost_From_The_Excess_Prosumer_Breaker=0;
    P1_C1_Excess_C1_Control=0;
end

%%Case 2 Discharge

if (Load> P_Real_Grid_C1) || P_Real_Grid_C1<100
    V_Consumer_Battery_Boost_Breaker_Grid=0;
    V_Consumer_Battery_Buck_Breaker_Grid=0;
    Grid_Battery_Switch=1; 
    H1_Battery_Discharge=1;
    Buck_From_The_Excess_Prosumer_Breaker=0;
    Boost_From_The_Excess_Prosumer_Breaker=0;
    P1_C1_Excess_C1_Control=0;
end

== matlab function PVHome/Subsystem6/Subsystem/MATLAB Function4 ==
  data: u input; y output
function y = fcn(u)
% This will output 1 - u
y = 1 - u;

== matlab function PVHome/Subsystem6/Subsystem/MATLAB Function9 ==
  data: Sixty input; V_Consumer_Batter input; Wind_Breaker_Boost_Signal_Out output
function Wind_Breaker_Boost_Signal_Out = fcn(Sixty, V_Consumer_Batter)
Sixty = abs(Sixty);
V_Consumer_Batter = abs(V_Consumer_Batter);

D=1-(Sixty/V_Consumer_Batter);
Wind_Breaker_Boost_Signal_Out = D; %Vout

== matlab function PVHome/Subsystem6/Subsystem/MATLAB Function1 ==
  data: u input; y output
function y = fcn(u)
% This will output 1 - u
y = 1 - u;

== matlab function PVHome/Subsystem6/Subsystem/MATLAB Function2 ==
  data: Sixty input; V_Consumer_Batter input; Wind_Breaker_Boost_Signal_Out output
function Wind_Breaker_Boost_Signal_Out = fcn(Sixty, V_Consumer_Batter)
Sixty = abs(Sixty);
V_Consumer_Batter = abs(V_Consumer_Batter);

D=1-(Sixty/V_Consumer_Batter);
Wind_Breaker_Boost_Signal_Out = D; %Vout

== matlab function PVHome/Subsystem5/Subsystem/MATLAB Function1 ==
  data: u input; y output
function y = fcn(u)
% This will output 1 - u
y = 1 - u;

== matlab function PVHome/Subsystem5/Subsystem/MATLAB Function2 ==
  data: Sixty input; V_Consumer_Batter input; Wind_Breaker_Boost_Signal_Out output
function Wind_Breaker_Boost_Signal_Out = fcn(Sixty, V_Consumer_Batter)
Sixty = abs(Sixty);
V_Consumer_Batter = abs(V_Consumer_Batter);

D=1-(Sixty/V_Consumer_Batter);
Wind_Breaker_Boost_Signal_Out = D; %Vout

== matlab function PVHome/Subsystem5/Subsystem/MATLAB Function4 ==
  data: u input; y output
function y = fcn(u)
% This will output 1 - u
y = 1 - u;

== matlab function PVHome/Subsystem5/Subsystem/MATLAB Function9 ==
  data: Sixty input; V_Consumer_Batter input; Wind_Breaker_Boost_Signal_Out output
function Wind_Breaker_Boost_Signal_Out = fcn(Sixty, V_Consumer_Batter)
Sixty = abs(Sixty);
V_Consumer_Batter = abs(V_Consumer_Batter);

D=1-(Sixty/V_Consumer_Batter);
Wind_Breaker_Boost_Signal_Out = D; %Vout

== matlab function PVHome/Subsystem4/Subsystem/MATLAB Function1 ==
  data: u input; y output
function y = fcn(u)
% This will output 1 - u
y = 1 - u;

== matlab function PVHome/Subsystem4/Subsystem/MATLAB Function2 ==
  data: Sixty input; V_Consumer_Batter input; Wind_Breaker_Boost_Signal_Out output
function Wind_Breaker_Boost_Signal_Out = fcn(Sixty, V_Consumer_Batter)
Sixty = abs(Sixty);
V_Consumer_Batter = abs(V_Consumer_Batter);

D=1-(Sixty/V_Consumer_Batter);
Wind_Breaker_Boost_Signal_Out = D; %Vout

== matlab function PVHome/Subsystem4/Subsystem/MATLAB Function4 ==
  data: u input; y output
function y = fcn(u)
% This will output 1 - u
y = 1 - u;
